simulink model "Propofol_Children_2016"  (R2022a)
settings: Solver=VariableStepAuto  StartTime=0.0  StopTime=100  FixedStep=1e-3  RelTol=1e-3
values from neighbouring files (symbols this model uses):
  delay = Patient(patient, 1)    [PlotME.m]
  E0 = Patient(patient, 5)    [PlotME.m]
  E50 = Patient(patient, 3)    [PlotME.m]
  gamma = Patient(patient, 4)    [PlotME.m]
  k = Patient(patient, 2)    [PlotME.m]
  Kp = zeros(1,size(Metodos,2))    [PID_Tuning.m]    (also in PI_Tuning.m; SinteseParam.m = tal/(K*(gama + atraso)))
  Td = zeros(1,size(Metodos,2))    [PID_Tuning.m]    (also in PI_Tuning.m)
  Ti = zeros(1,size(Metodos,2))    [PID_Tuning.m]    (also in PI_Tuning.m; SinteseParam.m = min(tal, 4*(atraso+gama)))
settings Model: Creator=mluser  LastModifiedBy=Cliente
settings SolverCC: AlgebraicLoopSolver=TrustRegion
settings DebuggingCC: SFMachineParentedDataDiag=warning  ArithmeticOperatorsInVariantConditions=warning
settings SFSimCC: CustomCodeUndefinedFunction=UseInterfaceOnly
settings RTWCC: DLArmComputeVersion=19.05
settings CodeAppCC: StateflowObjectComments=on

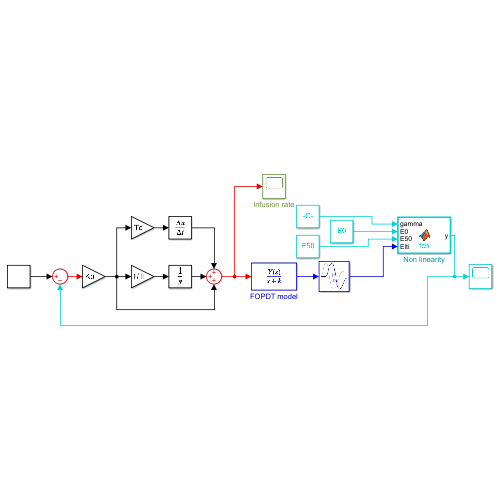
[thumbnail: Simulink's stored preview of the top-level diagram]
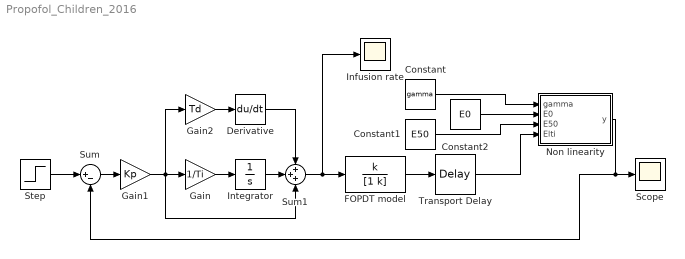
== system Propofol_Children_2016 ==
  Constant : Constant  Value=gamma
  Constant1 : Constant  Value=E50
  Constant2 : Constant  Value=E0
  Derivative : Derivative
  FOPDT model : TransferFcn  Numerator=k  Denominator=[1 k]
  Gain : Gain  Gain=1/Ti
  Gain1 : Gain  Gain=Kp
  Gain2 : Gain  Gain=Td
  Infusion rate : Scope
  Integrator : Integrator
  Non linearity : MATLAB Function  TreatAsAtomicUnit=on
  Scope : Scope
  Step : Step  Before=E0  After=50  SampleTime=0
  Sum : Sum  Inputs=|+-
  Sum1 : Sum  Inputs=+++
  Transport Delay : TransportDelay  DelayTime=delay/60
  wires:
  FOPDT model/1 -> Transport Delay/1
  Non linearity/1(y) -> Sum/2, Scope/1
  Step/1 -> Sum/1
  Constant2/1 -> Non linearity/2(E0)
  Constant1/1 -> Non linearity/3(E50)
  Constant/1 -> Non linearity/1(gamma)
  Transport Delay/1 -> Non linearity/4(Elti)
  Gain/1 -> Integrator/1
  Gain1/1 -> Gain2/1, Sum1/3, Gain/1
  Sum/1 -> Gain1/1
  Sum1/1 -> FOPDT model/1, Infusion rate/1
  Integrator/1 -> Sum1/2
  Gain2/1 -> Derivative/1
  Derivative/1 -> Sum1/1

== matlab function Propofol_Children_2016/Non linearity ==
  data: gamma input; y output; E0 input; E50 input; Elti input
function y = fcn(gamma,E0,E50,Elti)

y = E0-E0*Elti^gamma/(E50^gamma+Elti^gamma);
